simulink model "sgMdl_IO145_DMALoopback"  (R2024b)
settings: Solver=FixedStepAuto  StartTime=0.0  StopTime=inf  RelTol=1e-3  EnableMultiTasking=on
undefined symbols (not defined in the file): modelRate, moduleRate, sineFreq
libraries: speedgoatlib_IO145 x3, speedgoatlib_interrupt x1, dspsrcs4 x1
Description:
  | IO145 - DMA Loopback
settings Model: ModifiedByFormat=Speedgoat  SimulationMode=external  ExtModeTrigDuration=100000  Creator=Speedgoat  LastModifiedBy=Speedgoat
settings SolverCC: ConcurrentTasks=on  AlgebraicLoopSolver=TrustRegion  PositivePriorityOrder=on  InsertRTBMode=Never (minimum delay)
settings DataIOCC: SaveFormat=Array  SaveState=on  SignalLoggingName=logsOut
settings OptimizationCC: BlockReduction=off  BooleanDataType=off  OptimizeBlockIOStorage=off  BufferReuse=off  GlobalBufferReuse=off  ExpressionFolding=off  LocalBlockOutputs=off  InitFltsAndDblsToZero=on  OptimizeDataStoreBuffers=off  BusAssignmentInplaceUpdate=off
settings DebuggingCC: SaveWithParameterizedLinksMsg=none  UnderspecifiedInitializationDetection=Classic  MergeDetectMultiDrivingBlocksExec=none  CheckExecutionContextPreStartOutputMsg=on  SignalResolutionControl=TryResolveAllWithWarning  TasksWithSamePriorityMsg=none  UnconnectedInputMsg=warning  UnconnectedOutputMsg=warning  UnconnectedLineMsg=warning  SFUnexpectedBacktrackingDiag=warning  SFNoUnconditionalDefaultTransitionDiag=warning  SFExecutionAtInitializationDiag=none  ArithmeticOperatorsInVariantConditions=warning
settings HardwareCC: ProdBitPerLong=64  ProdLongLongMode=on  ProdHWDeviceType=Intel->x86-64 (Linux 64)
settings ModelReferenceCC: EnableRefExpFcnMdlSchedulingChecks=on  PropagateSignalLabelsOutOfModel=off
settings SFSimCC: SimUseLocalCustomCode=off  SimTargetLang=C++
settings RTWCC: Description=Speedgoat Real-Time Target Machine  SystemTargetFile=speedgoat.tlc  TemplateMakefile=slrealtime_default_tmf  RTWUseLocalCustomCode=off  Toolchain=Simulink Real-Time Toolchain  BuildConfiguration=Faster Runs  TargetLang=C++  GPUComputeCapability=3.5  DLArmComputeVersion=19.05
settings CodeAppCC: StateflowObjectComments=on
settings SimulinkRealTimeTargetCC: SubcomponentCodeInterfacePackaging=Reusable function  MATLABClassNameForMDSCustomization=Simulink.SoftwareTarget.GRTCustomization  InstructionSetFMA=off  LogToMDFFile=off  SLRTFileLogMaxRuns=10
settings ConfigComp: CovMetricSettings=dw  CovSaveCumulativeToWorkspaceVar=on  CovSaveSingleToWorkspaceVar=on  CovExternalEMLEnable=off  CovSFcnEnable=off  CovBoundaryAbsTol=1.0e-5

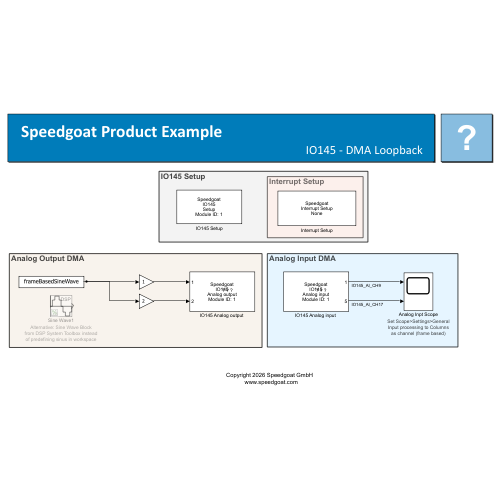
[thumbnail: Simulink's stored preview of the top-level diagram]
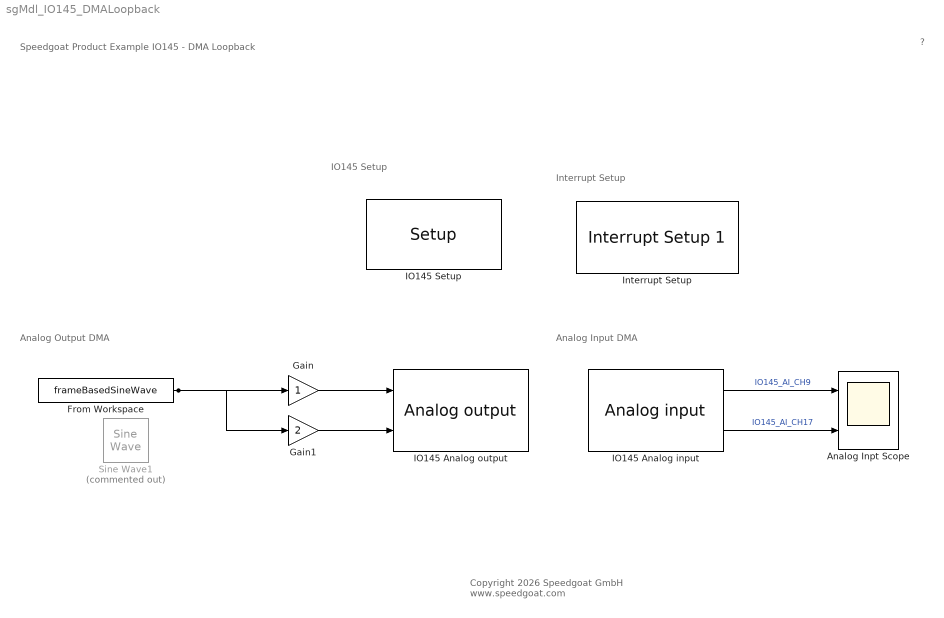
== system sgMdl_IO145_DMALoopback ==
  note: Analog Input DMA
  note: Analog Output DMA
  note: Interrupt Setup
  note: IO145 Setup
  note: Speedgoat Product Example
      | IO145 - DMA Loopback
  note: ?
  note: Copyright 2026 Speedgoat GmbH
      |  www.speedgoat.com
  Analog Inpt Scope : Scope  NumInputPorts=2
      settings: AttributesFormatString=|
      | Set Scope>Settings>General
      | Input processing to Columns
      | as channel (frame based)
  From Workspace : FromWorkspace  VariableName=frameBasedSineWave  SampleTime=modelRate  Interpolate=off  OutputAfterFinalValue=Setting to zero
  Gain : Gain
  Gain1 : Gain  Gain=2
  "IO145 Analog input " : speedgoatlib_IO145/Analog input   parModuleId=1  parSampleTime=modelRate  parPciSlot=-1  parAdcChannels=[17 25]  parAdcNumActiveChannels=[0 0 1 1]  parAdcVoltageRange=[1 1 1 1 1 1 1 1 1 1 1 1 1 1 1 1 1 1 1 1 1 1 1 1 1 1 1 1 1 1 1 1]  parAdcCoupling=[1 1 1 1]  parAdcContSampling=0  parAdcDmaEnable=1  parAdcActiveDmaDevices=[1 1 1 1]  parAdcFrameSize=5
      settings: SourceProductName=IO145
  "IO145 Analog output " : speedgoatlib_IO145/Analog output   parModuleId=1  parSampleTime=-1  parPciSlot=-1  parDacChannels=[3 4]  parDacVoltageRange=[1 1 7 7 7 7 1 1]  parDacOverRange=[0 0 0 0 0 0 0 0]  parDacInitValues=[0 0]  parDacReset=[1 1]  parDacSyncOut=1  parDacDmaEnable=1  parDacActiveDmaDevices=[1 1 1 1]  parDacDmaLatency=2  parDacFrameSize=5
      settings: SourceProductName=IO145
  IO145 Setup : speedgoatlib_IO145/Setup   parPciSlot=-1  parModuleId=1  parInterModuleSync=Independent  parConvClockBaseRate=20MHz  parConvClock1Divider=4000  parConvClock2Divider=20000  parFrameTriggerEnable=off  parFrameTriggerDivider=10  parConvClock1BaseRate=1  parConvClock2BaseRate=1  parFrameTriggerClock=1  parAdcCoupling1=Differential  parAdcChannels1=[1 2]  parAdcChannel11=off  parAdcChannel12=off  parAdcChannel13=off  parAdcChannel14=off  parAdcChannel15=off  parAdcChannel16=off  parAdcChannel17=off  parAdcChannel18=off  parAdcRangeAll1=+-25 mA  parVoltageRangePerChannelEn1=off  parAdcRange11=+-25 mA  parAdcRange12=+-25 mA  parAdcRange13=+-25 mA  parAdcRange14=+-25 mA  parAdcRange15=+-25 mA  parAdcRange16=+-25 mA  parAdcRange17=+-25 mA  parAdcRange18=+-25 mA  parAdcCoupling2=Differential  parAdcChannels2=[9 10]  parAdcChannel21=off  parAdcChannel22=off  parAdcChannel23=off  parAdcChannel24=off  parAdcChannel25=off  parAdcChannel26=off  parAdcChannel27=off  parAdcChannel28=off  parAdcRangeAll2=+-25 mA  parVoltageRangePerChannelEn2=off  parAdcRange21=+-25 mA  parAdcRange22=+-25 mA  parAdcRange23=+-25 mA  parAdcRange24=+-25 mA  parAdcRange25=+-25 mA  parAdcRange26=+-25 mA  parAdcRange27=+-25 mA  parAdcRange28=+-25 mA  parAdcCoupling3=Differential  parAdcChannels3=[17 18]  parAdcChannel31=on  parAdcChannel32=off  parAdcChannel33=off  parAdcChannel34=off  parAdcChannel35=off  parAdcChannel36=off  parAdcChannel37=off  parAdcChannel38=off  parAdcRangeAll3=+-10V  parVoltageRangePerChannelEn3=off  parAdcRange31=+-10V  parAdcRange32=+-10V  parAdcRange33=+-10V  parAdcRange34=+-10V  parAdcRange35=+-10V  parAdcRange36=+-10V  parAdcRange37=+-10V  parAdcRange38=+-10V  parAdcCoupling4=Differential  parAdcChannels4=[25 26]  parAdcChannel41=on  parAdcChannel42=off  parAdcChannel43=off  parAdcChannel44=off  parAdcChannel45=off  parAdcChannel46=off  parAdcChannel47=off  parAdcChannel48=off  parAdcRangeAll4=+-10V  parVoltageRangePerChannelEn4=off  parAdcRange41=+-10V  parAdcRange42=+-10V  parAdcRange43=+-10V  parAdcRange44=+-10V  parAdcRange45=+-10V  parAdcRange46=+-10V  parAdcRange47=+-10V  parAdcRange48=+-10V  parAdcChannels=[17 25]  parAdcNumActiveChannels=[0 0 1 1]  parAdcVoltageRange=[1 1 1 1 1 1 1 1 1 1 1 1 1 1 1 1 1 1 1 1 1 1 1 1 1 1 1 1 1 1 1 1]  parAdcCoupling=[1 1 1 1]  parAdcContSampling=off  parAdcAutoCorrection=on  parAdcDmaEnable=on  parAdcDmaClock=Clock 1  parAdcFrameSize_=frameSize  parAdcSampleTime_=-1  parAdcActiveDmaDevices=[1 1 1 1]  parAdcFrameTriggerEnable=0  parAdcFrameSize=5  parAdcSampleTime=0.001  parDacChannels=[1 2 3 4]  parDacChannel1=off  parDacChannel2=off  parDacChannel3=on  parDacChannel4=on  parDacChannel5=off  parDacChannel6=off  parDacChannel7=off  parDacChannel8=off  parDacInitValues=0  parDacResets=1  parDacVoltageRange=[1 1 7 7 7 7 1 1]  parDacOverRange=[0 0 0 0 0 0 0 0]  parDacRange1=0-5 V  parDacInitValue1=0  parDacReset1=on  parDacRange2=0-5 V  parDacInitValue2=0  parDacReset2=on  parDacRange3=+-10 V  parDacInitValue3=0  parDacReset3=on  parDacRange4=+-10 V  parDacInitValue4=0  parDacReset4=on  parDacRange5=+-10 V  parDacInitValue5=0  parDacReset5=on  parDacRange6=+-10 V  parDacInitValue6=0  parDacReset6=on  parDacRange7=0-5 V  parDacInitValue7=0  parDacReset7=on  parDacRange8=0-5 V  parDacInitValue8=0  parDacReset8=on  parDacAutoCorrection=on  parDacSyncOut=on  parDacDmaEnable=on  parDacDmaLatency=Until next frame  parDacDmaClock=Clock 1  parDacFrameSize_=frameSize  parDacSampleTime_=-1  parDacActiveDmaDevices=[1 1 1 1]  parDacFrameTriggerEnable=0  parDacFrameSize=5  parDacSampleTime=0.001  parDiChannels=[1 2 3 4]  parDoChannels=[5 6 7 8]  parDioChannel1=In  parDioChannel2=In  parDioChannel3=In  parDioChannel4=In  parDioChannel5=Out  parDioChannel6=Out  parDioChannel7=Out  parDioChannel8=Out  parDoInitValues=[0 0 0 0]  parDoReset=[1 1 1 1]  parDoInitValue1=0  parDoReset1=on  parDoInitValue2=0  parDoReset2=on  parDoInitValue3=0  parDoReset3=on  parDoInitValue4=0  parDoReset4=on  parDoInitValue5=0  parDoReset5=on  parDoInitValue6=0  parDoReset6=on  parDoInitValue7=0  parDoReset7=on  parDoInitValue8=0  parDoReset8=on  parDiDebounceEnable=off  parDiDebounceTime=0  parDiDebounceValue=0  parDioPullRefFront=Floating  parDioPullRefRear=Floating
      settings: SourceProductName=IO145
  Interrupt Setup : speedgoatlib_interrupt/Interrupt Setup 1  parModuleTrigger=on  parPollingMode=off  parPriorityConf=High  parPriority=241  confStartFcn=IO145_start_public  confStopFcn=IO145_stop_public  confIsrFcn=IO145_isr_public  confMapFcn=IO145_map_public  confHookFile=io145_int_hooks.c  confIrqNr=-1  confIsPolling=off  confModID=16776961  confSelectedInt=Speedgoat IO145 DMA interrupt  confSelectedId=1  confSelectedChannel=[]  confData=254  confForcePollingMode=off
  Sine Wave1 : dspsrcs4/Sine Wave  Commented=on  Amplitude=1  Frequency=sineFreq  Phase=0  SampleMode=Discrete  OutComplex=Real  CompMethod=Table lookup  TableSize=Speed  SampleTime=1/moduleRate  SamplesPerFrame=frameSize  ResetState=Restart at time zero  OutputFrames=off  dataType=double  wordLen=16  udDataType=sfix(16)  fracBitsMode=Best precision  numFracBits=15  OutDataTypeStr=double  LastOutDataTypeStr=double
      settings: AttributesFormatString=|
      | Alternative: Sine Wave Block
      | from DSP System Toolbox instead
      | of predefining sinus in workspace
  wires:
  Gain/1 -> "IO145 Analog output "/1
  Gain1/1 -> "IO145 Analog output "/2
  From Workspace/1 -> Gain1/1, Gain/1
  "IO145 Analog input "/1 -> Analog Inpt Scope/1  "IO145_AI_CH9"
  "IO145 Analog input "/2 -> Analog Inpt Scope/2  "IO145_AI_CH17"
